simulink model "PID_method"  (R2018b)
settings: Solver=FixedStepAuto  StartTime=0.0  StopTime=inf  FixedStep=TS  RelTol=1e-3  EnableMultiTasking=on
values from neighbouring files (symbols this model uses):
  ES = -C2DEG*D2R    (= -0.00872664625997)    [parameter.m]
  GS = GyroS*D2R    [parameter.m]
  r_w = 0.016    [final.m]    (also in parameter.m)
  TS = 0.005    [parameter.m]
  tstart = .6    (= 0.6)    [parameter.m]
undefined symbols (not defined in the file or in its folder): DiscIntNeverNeededParam
libraries: simulink x2, arduinolib x2
settings Model: SimulationMode=external  ExtModeTrigDuration=2  Creator=luyey  LastModifiedBy=luyey
settings OptimizationCC: EnhancedBackFolding=on  PassReuseOutputArgsAs=Individual arguments  MaxStackSize=64  OptimizeBlockOrder=speed  DifferentSizesBufferReuse=on  OptimizationCustomize=off
settings DebuggingCC: ParameterTunabilityLossMsg=error
settings HardwareCC: ProdBitPerInt=16  ProdBitPerPointer=16  ProdBitPerSizeT=16  ProdBitPerPtrDiffT=16  ProdLargestAtomicFloat=None  ProdWordSize=8  ProdHWDeviceType=Atmel->AVR  UseEmbeddedCoderFeatures=off  UseSimulinkCoderFeatures=off
settings SFSimCC: MATLABDynamicMemAlloc=off
settings RTWCC: SystemTargetFile=ert.tlc  HardwareBoard=Arduino Mega 2560  TemplateMakefile=ert_default_tmf  GenerateReport=on  Toolchain=Arduino AVR  BuildConfiguration=Faster Runs  IncludeHyperlinkInReport=on  LaunchReport=on  GenerateTraceInfo=on  GenerateTraceReport=on  GenerateTraceReportSl=on  GenerateTraceReportSf=on  GenerateTraceReportEml=on
settings CodeAppCC: ForceParamTrailComments=on  IgnoreCustomStorageClasses=off  OperatorAnnotations=on  SimulinkDataObjDesc=on  SFDataObjDesc=on  MangleLength=10  InsertBlockDesc=on
settings ERTTargetCC: SupportContinuousTime=on  SupportNonInlinedSFcns=on  SupportVariableSizeSignals=on

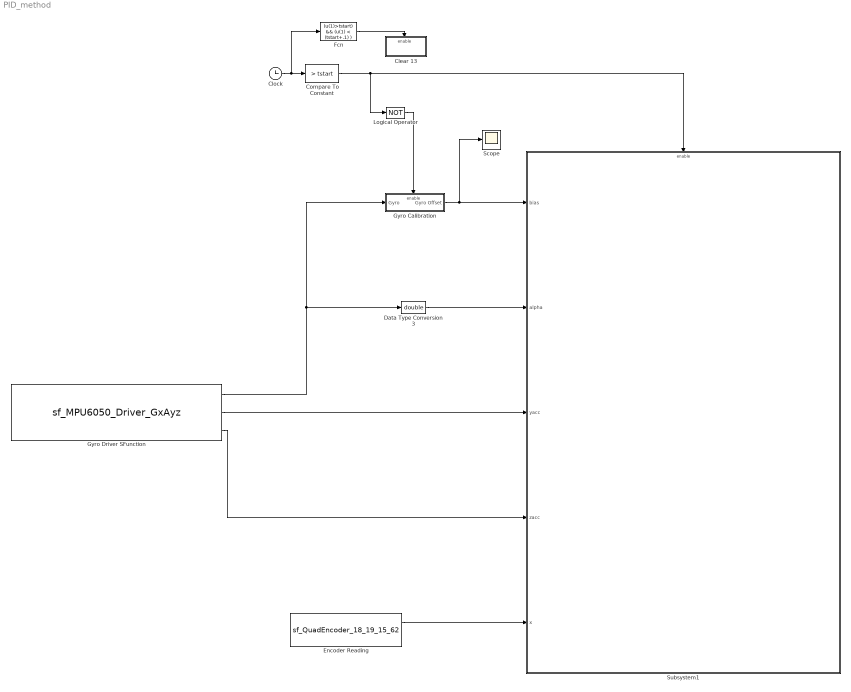
== system PID_method ==
  "Clear 13 " : Subsystem  TreatAsAtomicUnit=on
  Clock : Clock
  Compare To Constant : simulink/Logic and Bit Operations/Compare To Constant  relop=>  const=tstart  OutDataTypeStr=boolean
  Data Type Conversion3 : DataTypeConversion  OutDataTypeStr=double
  Encoder Reading : S-Function  InitFcn=try, set_param(gcb,'FunctionName','sf_QuadEncoder_18_19_15_62'), end  FunctionName=sf_QuadEncoder_18_19_15_62  Parameters=uint8([0 1]),uint8([18 62]),uint8([19 15])  SFunctionModules=sf_QuadEncoder_18_19_15_62_wrapper  SFunctionDeploymentMode=off  EnableBusSupport=off  mask(S-Function Builder){}
      mask init:
      | val = [[.9  0.75 0.75 1 1 .9 .9 1]',[1 1 0.75 0.75 .9 .9 1 .9]'];try , sys = get_param(gcb,'SfunBuilderFcnName');if isempty(sys), sys = get_param(gcb,'FunctionName'); end,catch, sys = get_param(gcb,'FunctionName'); end
      settings: CopyFcn=set_param(gcbh,'LinkStatus','none')  PreSaveFcn=try, set_param(gcb,'FunctionName','sf_QuadEncoder_18_19_15_62'), end  OpenFcn=sfunctionwizard(gcbh)
      mask Display: plot(val(:,1),val(:,2)),disp(sys), port_label('output',1,'pos1'), port_label('output',2,'pos2')
  Fcn : Fcn  Expr=(u(1)>tstart) && (u(1) < (tstart+.1) )
  Gyro Calibration : Subsystem  TreatAsAtomicUnit=on
  Gyro Driver SFunction : S-Function  InitFcn=try, set_param(gcb,'FunctionName','sf_MPU6050_Driver_GxAyz'), end  FunctionName=sf_MPU6050_Driver_GxAyz  SFunctionModules=sf_MPU6050_Driver_GxAyz_wrapper  SFunctionDeploymentMode=off  EnableBusSupport=off  mask(S-Function Builder){}
      mask help: Simulink:masks:SFunctionBuilder_MD
      mask init: same as PID_method/Encoder Reading
      settings: CopyFcn=set_param(gcbh,'LinkStatus','none')  PreSaveFcn=try, set_param(gcb,'FunctionName','sf_MPU6050_Driver_GxAyz'), end  OpenFcn=sfunctionwizard(gcbh)
      mask Display: plot(val(:,1),val(:,2)),disp(sys), port_label('output',1,'x_vel'), port_label('output',2,'y_acc'), port_label('output',3,'z_acc')
  Logical Operator : Logic  Operator=NOT  AllPortsSameDT=off  OutDataTypeStr=boolean
  Scope : Scope
  Subsystem1 : Subsystem
  wires:
  Data Type Conversion3/1 -> Subsystem1/2(alpha)
  Gyro Driver SFunction/2 -> Subsystem1/3(yacc)
  Gyro Driver SFunction/3 -> Subsystem1/4(zacc)
  Encoder Reading/1 -> Subsystem1/5(x)
  Fcn/1 -> "Clear 13 "/Enable
  Gyro Driver SFunction/1 -> Gyro Calibration/1(Gyro), Data Type Conversion3/1
  Clock/1 -> Fcn/1, Compare To Constant/1
  Compare To Constant/1 -> Subsystem1/Enable, Logical Operator/1
  Logical Operator/1 -> Gyro Calibration/Enable
  Gyro Calibration/1(Gyro Offset) -> Scope/1, Subsystem1/1(bias)

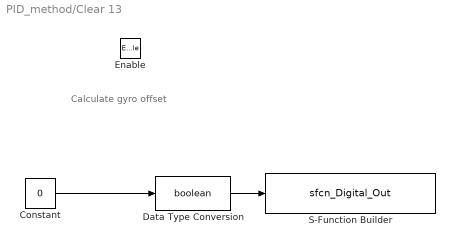
== system PID_method/Clear 13  ==
  note: Calculate gyro offset
  Enable : EnablePort
  Constant : Constant  Value=0
  Data Type Conversion : DataTypeConversion  OutDataTypeStr=boolean
  S-Function Builder : S-Function  InitFcn=try, set_param(gcb,'FunctionName','sfcn_Digital_Out'), end  FunctionName=sfcn_Digital_Out  Parameters=uint8(13)  SFunctionModules=sfcn_Digital_Out_wrapper  SFunctionDeploymentMode=off  EnableBusSupport=off  mask(S-Function Builder){}
      mask init: same as PID_method/Encoder Reading
      settings: CopyFcn=set_param(gcbh,'LinkStatus','none')  PreSaveFcn=try, set_param(gcb,'FunctionName','sfcn_Digital_Out'), end  OpenFcn=sfunctionwizard(gcbh)
      mask Display: plot(val(:,1),val(:,2)),disp(sys), port_label('input',1,'in')
  wires:
  Data Type Conversion/1 -> S-Function Builder/1
  Constant/1 -> Data Type Conversion/1

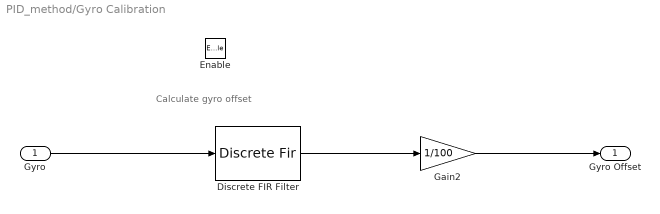
== system PID_method/Gyro Calibration ==
  note: Calculate gyro offset
  Gyro : Inport
  Enable : EnablePort
  Discrete FIR Filter : DiscreteFir  Coefficients=ones(1,100)
  Gain2 : Gain  Gain=1/100  OutDataTypeStr=Inherit: Same as input  ParamDataTypeStr=Inherit: Same as input
  Gyro Offset : Outport
  wires:
  Gyro/1 -> Discrete FIR Filter/1
  Discrete FIR Filter/1 -> Gain2/1
  Gain2/1 -> Gyro Offset/1

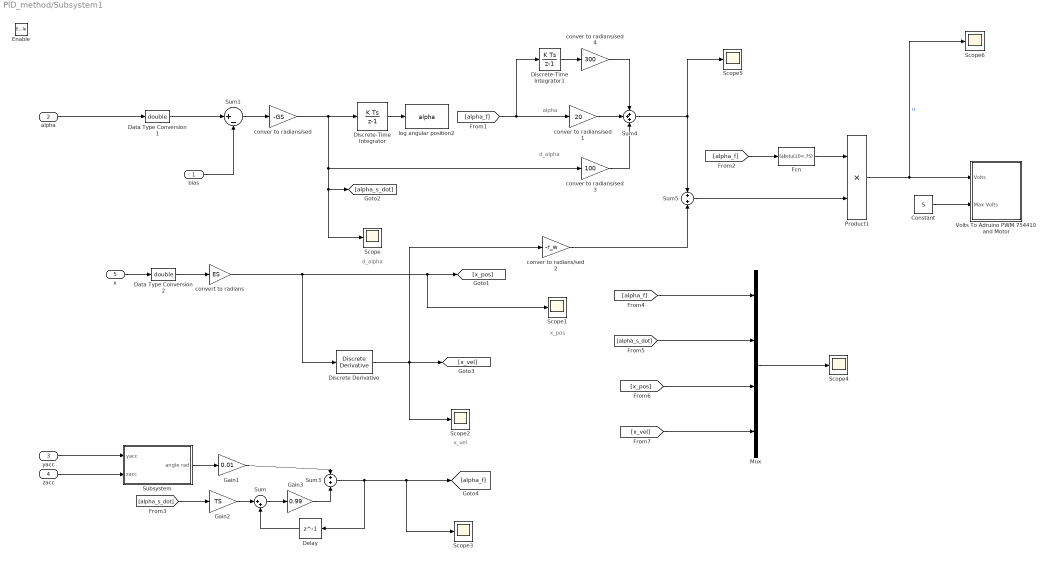
== system PID_method/Subsystem1 ==
  note: alpha
  note: d_alpha
  note: d_alpha
  note: x_pos
  note: x_vel
  bias : Inport
  alpha : Inport  Port=2
  yacc : Inport  Port=3
  zacc : Inport  Port=4
  x : Inport  Port=5
  Enable : EnablePort
  Constant : Constant  Value=5
  Data Type Conversion1 : DataTypeConversion  OutDataTypeStr=double
  Data Type Conversion2 : DataTypeConversion  OutDataTypeStr=double
  Delay : Delay  DelayLength=1  InitialCondition=0
  Discrete Derivative : simulink/Discrete/Discrete Derivative  gainval=1.0  ICPrevScaledInput=0.0  OutMin=[]  OutMax=[]  OutDataType=fixdt(1, 16)  OutScaling=2^-10  DoSatur=off
  Discrete-Time Integrator : DiscreteIntegrator  SampleTime=TS  ICPrevOutput=DiscIntNeverNeededParam  ICPrevScaledInput=DiscIntNeverNeededParam
  Discrete-Time Integrator1 : DiscreteIntegrator  SampleTime=-1  LimitOutput=on  UpperSaturationLimit=3/374  LowerSaturationLimit=-3/374  ICPrevOutput=DiscIntNeverNeededParam  ICPrevScaledInput=DiscIntNeverNeededParam
  Fcn : Fcn  Expr=(abs(u(1))<.75)
  Gain1 : Gain  Gain=0.01
  Gain2 : Gain  Gain=TS
  Gain3 : Gain  Gain=0.99
  Mux : Mux
  Product1 : Product  RndMeth=Zero
  Scope{,1..6} (7 alike) : Scope
  Subsystem : Subsystem
  Sum : Sum  Inputs=|++
  Sum1 : Sum  Inputs=|+-
  Sum3 : Sum
  Sum4 : Sum  Inputs=+++
  Sum5 : Sum
  Volts To Adruino PWM 754410 and Motor : Subsystem
  conver to radians/sed : Gain  Gain=-GS
  conver to radians/sed1 : Gain  Gain=20
  conver to radians/sed2 : Gain  Gain=-r_w
  conver to radians/sed3 : Gain  Gain=100
  conver to radians/sed4 : Gain  Gain=300
  convert to radians : Gain  Gain=ES  OutDataTypeStr=double
  log angular position2 : ToWorkspace  VariableName=alpha  SampleTime=-1
  wires:
  Gain3/1 -> Sum3/2
  conver to radians/sed/1 -> conver to radians/sed3/1, [alpha_s_dot], Scope/1, Discrete-Time Integrator/1
  Gain2/1 -> Sum/1
  convert to radians/1 -> Discrete Derivative/1, [x_pos], Scope1/1
  [alpha_f] -> conver to radians/sed1/1, Discrete-Time Integrator1/1
  conver to radians/sed4/1 -> Sum4/1
  alpha/1 -> Data Type Conversion1/1
  zacc/1 -> Subsystem/2(zacc)
  conver to radians/sed1/1 -> Sum4/2
  yacc/1 -> Subsystem/1(yacc)
  Data Type Conversion2/1 -> convert to radians/1
  Sum3/1 -> Scope3/1, [alpha_f], Delay/1
  conver to radians/sed3/1 -> Sum4/3
  Fcn/1 -> Product1/1
  bias/1 -> Sum1/2
  Discrete Derivative/1 -> [x_vel], conver to radians/sed2/1, Scope2/1
  Sum4/1 -> Sum5/1, Scope5/1
  Sum5/1 -> Product1/2
  [alpha_f] -> Fcn/1
  Data Type Conversion1/1 -> Sum1/1
  Delay/1 -> Sum/2
  Sum1/1 -> conver to radians/sed/1
  x/1 -> Data Type Conversion2/1
  conver to radians/sed2/1 -> Sum5/2
  Sum/1 -> Gain3/1
  Gain1/1 -> Sum3/1
  Subsystem/1(angle rad) -> Gain1/1
  Discrete-Time Integrator1/1 -> conver to radians/sed4/1
  [alpha_s_dot] -> Gain2/1
  Discrete-Time Integrator/1 -> log angular position2/1
  Mux/1 -> Scope4/1
  [alpha_f] -> Mux/1
  [alpha_s_dot] -> Mux/2
  [x_pos] -> Mux/3
  [x_vel] -> Mux/4
  Product1/1 -> Volts To Adruino PWM 754410 and Motor/1(Volts), Scope6/1  "u"
  Constant/1 -> Volts To Adruino PWM 754410 and Motor/2(Max Volts)

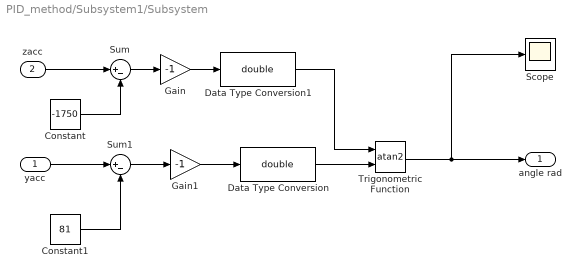
== system PID_method/Subsystem1/Subsystem ==
  yacc : Inport
  zacc : Inport  Port=2
  Constant : Constant  Value=-1750
  Constant1 : Constant  Value=81
  Data Type Conversion : DataTypeConversion  OutDataTypeStr=double
  Data Type Conversion1 : DataTypeConversion  OutDataTypeStr=double
  Gain : Gain  Gain=-1
  Gain1 : Gain  Gain=-1
  Scope : Scope
  Sum : Sum  Inputs=|+-
  Sum1 : Sum  Inputs=|+-
  Trigonometric Function : Trigonometry  Operator=atan2
  angle rad : Outport
  wires:
  Trigonometric Function/1 -> Scope/1, angle rad/1
  Data Type Conversion1/1 -> Trigonometric Function/1
  Data Type Conversion/1 -> Trigonometric Function/2
  zacc/1 -> Sum/1
  yacc/1 -> Sum1/1
  Constant/1 -> Sum/2
  Constant1/1 -> Sum1/2
  Sum/1 -> Gain/1
  Gain/1 -> Data Type Conversion1/1
  Sum1/1 -> Gain1/1
  Gain1/1 -> Data Type Conversion/1

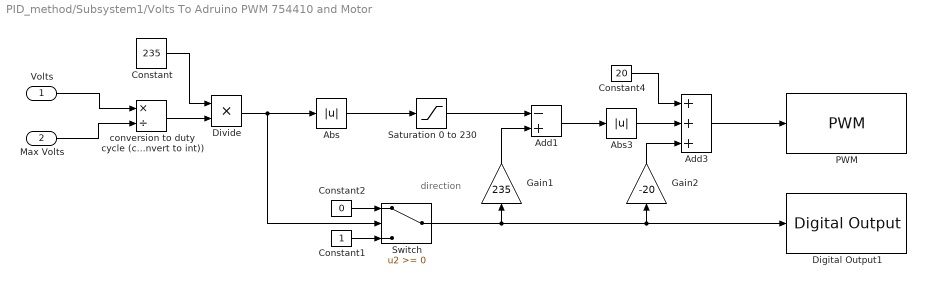
== system PID_method/Subsystem1/Volts To Adruino PWM 754410 and Motor ==
  note: direction
  Volts : Inport
  Max Volts : Inport  Port=2
  Abs : Abs
  Abs3 : Abs
  Add1 : Sum  Inputs=-+
  Add3 : Sum  Inputs=+++
  Constant : Constant  Value=235
  Constant1 : Constant
  Constant2 : Constant  Value=0
  Constant4 : Constant  Value=20
  Digital Output1 : arduinolib/Digital Output  pinNumber=6  blockPlatform=arduino
  Divide : Product  Inputs=**
  Gain1 : Gain  Gain=235
  Gain2 : Gain  Gain=-20
  PWM : arduinolib/PWM  pinNumber=8  EnableInputFrequency=off  InitialFrequency=2000  InitialDutyCycle=0  NotificationType=None  blockPlatform=arduino
  Saturation 0 to 230 : Saturate  UpperLimit=230  LowerLimit=0
  Switch : Switch
  conversion to duty cycle (convert to int)) : Product  Inputs=*/  OutDataTypeStr=double
  wires:
  Max Volts/1 -> conversion to duty cycle (convert to int))/2
  Abs3/1 -> Add3/2
  Constant4/1 -> Add3/1
  Volts/1 -> conversion to duty cycle (convert to int))/1
  Abs/1 -> Saturation 0 to 230/1
  Add1/1 -> Abs3/1
  Constant/1 -> Divide/1
  Saturation 0 to 230/1 -> Add1/1
  Gain1/1 -> Add1/2
  Constant2/1 -> Switch/1
  Gain2/1 -> Add3/3
  Switch/1 -> Gain1/1, Gain2/1, Digital Output1/1
  Divide/1 -> Switch/2, Abs/1
  Add3/1 -> PWM/1
  Constant1/1 -> Switch/3
  conversion to duty cycle (convert to int))/1 -> Divide/2
